simulink model "TP1_simulink"  (R2024a)
settings: Solver=ode4  StartTime=0.0  StopTime=4200  FixedStep=0.1  RelTol=1e-3
values from neighbouring files (symbols this model uses):
  h_eq = 0.45    [TP1.m]
  Qi = 0.000133333    [TP1.m]
  u_eq = Qi/(sqrt(2*g*h_eq)*A)    [TP1.m]
libraries: cstblocks x4
settings Model: Creator=nicoh  LastModifiedBy=aguse
settings SolverCC: AlgebraicLoopSolver=TrustRegion
settings DataIOCC: ReturnWorkspaceOutputs=off
settings OptimizationCC: LifeSpan=inf
settings DebuggingCC: UnconnectedInputMsg=warning  UnconnectedOutputMsg=warning  UnconnectedLineMsg=warning  SFExecutionAtInitializationDiag=none  ArithmeticOperatorsInVariantConditions=warning
settings ModelReferenceCC: EnableRefExpFcnMdlSchedulingChecks=on
settings SFSimCC: SimUseLocalCustomCode=off  CustomCodeUndefinedFunction=UseInterfaceOnly
settings RTWCC: RTWUseLocalCustomCode=off  GPUComputeCapability=3.5  DLArmComputeVersion=19.05
settings CodeAppCC: StateflowObjectComments=on

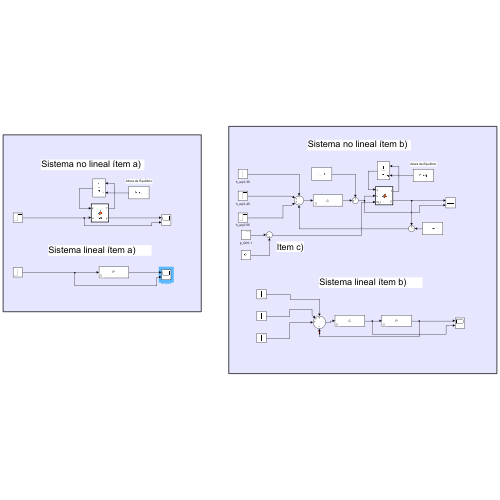
[thumbnail: Simulink's stored preview of the top-level diagram]
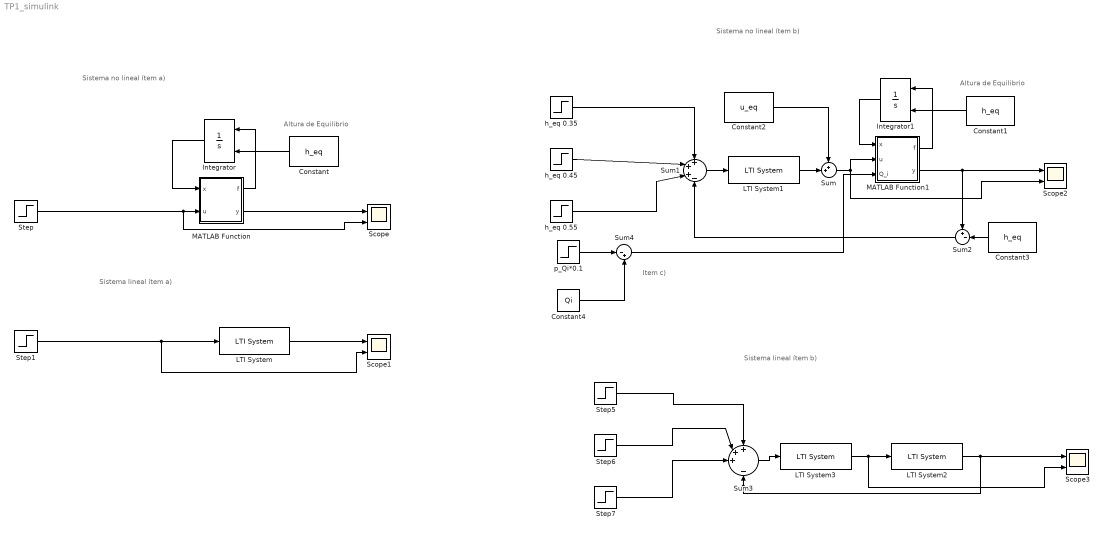
== system TP1_simulink ==
  note: Item c)
  note: Sistema no lineal ítem a)
  note: Altura de Equilibrio
  note: Sistema lineal ítem a)
  note: Altura de Equilibrio
  note: Sistema no lineal ítem b)
  note: Sistema lineal ítem b)
  Constant : Constant  Value=h_eq
  Constant1 : Constant  Value=h_eq
  Constant2 : Constant  Value=u_eq
  Constant3 : Constant  Value=h_eq
  Constant4 : Constant  Value=Qi
  Integrator : Integrator  InitialConditionSource=external
  Integrator1 : Integrator  InitialConditionSource=external
  LTI System : cstblocks/LTI System  sys=P  IC=[]  PadeOrder=0
  LTI System1 : cstblocks/LTI System  sys=C  IC=[]  PadeOrder=0
  LTI System2 : cstblocks/LTI System  sys=P  IC=[]  PadeOrder=0
  LTI System3 : cstblocks/LTI System  sys=C  IC=[]  PadeOrder=0
  MATLAB Function : MATLAB Function  TreatAsAtomicUnit=on
  MATLAB Function1 : MATLAB Function  TreatAsAtomicUnit=on
  Scope{,1..3} (4 alike) : Scope  NumInputPorts=2
  Step : Step  Time=120  Before=u_eq  After=1.1*u_eq  SampleTime=0
  Step1 : Step  Time=120  Before=u_eq  After=1.1*u_eq  SampleTime=0
  Step5 : Step  Time=60  After=-0.1  SampleTime=0
  Step6 : Step  Time=1200  After=0.1  SampleTime=0
  Step7 : Step  Time=2400  After=0.1  SampleTime=0
  Sum : Sum  Inputs=++|
  Sum1 : Sum  Inputs=+++-
  Sum2 : Sum  Inputs=+-|
  Sum3 : Sum  Inputs=+++|-
  Sum4 : Sum  Inputs=|-+
  h_eq 0.35 : Step  Time=60  After=-0.1  SampleTime=0
  h_eq 0.45 : Step  Time=1200  After=0.1  SampleTime=0
  h_eq 0.55 : Step  Time=2400  After=0.1  SampleTime=0
  p_Qi*0.1 : Step  Time=3500  After=0.1*Qi  SampleTime=0
  wires:
  Integrator/1 -> MATLAB Function/1(x)
  MATLAB Function/1(f) -> Integrator/1
  Constant/1 -> Integrator/2
  MATLAB Function/2(y) -> Scope/1
  Step/1 -> Scope/2, MATLAB Function/2(u)
  Step1/1 -> Scope1/2, LTI System/1
  Integrator1/1 -> MATLAB Function1/1(x)
  h_eq 0.35/1 -> Sum1/1
  MATLAB Function1/1(f) -> Integrator1/1
  MATLAB Function1/2(y) -> Scope2/1, Sum2/1
  Constant1/1 -> Integrator1/2
  LTI System1/1 -> Sum/2
  Sum/1 -> Scope2/2, MATLAB Function1/2(u)
  Constant2/1 -> Sum/1
  Sum1/1 -> LTI System1/1
  Constant3/1 -> Sum2/2
  Sum2/1 -> Sum1/4
  h_eq 0.45/1 -> Sum1/2
  h_eq 0.55/1 -> Sum1/3
  LTI System2/1 -> Sum3/4, Scope3/1
  LTI System3/1 -> Scope3/2, LTI System2/1
  Step7/1 -> Sum3/3
  Step5/1 -> Sum3/1
  Step6/1 -> Sum3/2
  Sum3/1 -> LTI System3/1
  Sum4/1 -> MATLAB Function1/3(Q_i)
  p_Qi*0.1/1 -> Sum4/1
  Constant4/1 -> Sum4/2
  LTI System/1 -> Scope1/1

== matlab function TP1_simulink/MATLAB Function1 ==
  data: x input; u input; f output; y output; Q_i input
function [f,y] = fcn(x,u,Q_i)
%Qi=0.000133333;
d=10.65e-3;
l_inf=10e-2;
l_sup=40e-2;
L=0.9;
g=9.8;
A=(pi/4)*d.^2;

f1=(Q_i-sqrt(2*g*x(1))*u*A)/(l_inf^2+2*l_inf*(l_sup-l_inf)*x(1)+(l_sup-l_inf)^2/L*x(1));
f=[f1];

y=x(1);

== matlab function TP1_simulink/MATLAB Function ==
  data: x input; u input; f output; y output
function [f,y] = fcn(x,u)
Qi=0.000133333;
d=10.65e-3;
l_inf=10e-2;
l_sup=40e-2;
L=0.9;
g=9.8;
A=(pi/4)*d.^2;

f1=(Qi-sqrt(2*g*x(1))*u*A)/(l_inf^2+2*l_inf*(l_sup-l_inf)*x(1)+(l_sup-l_inf)^2/L*x(1));
f=[f1];

y=x(1);
